simulink model "control_diagram_simple"  (R2018a)
settings: Solver=VariableStepAuto  StartTime=0.0  StopTime=10.0  RelTol=1e-3
libraries: fuzblock x2
settings Model: Creator=root  LastModifiedBy=User
settings DebuggingCC: LibraryContextMissingDiagnostic=warning
settings SFSimCC: SimUseLocalCustomCode=on
settings RTWCC: RTWUseLocalCustomCode=on

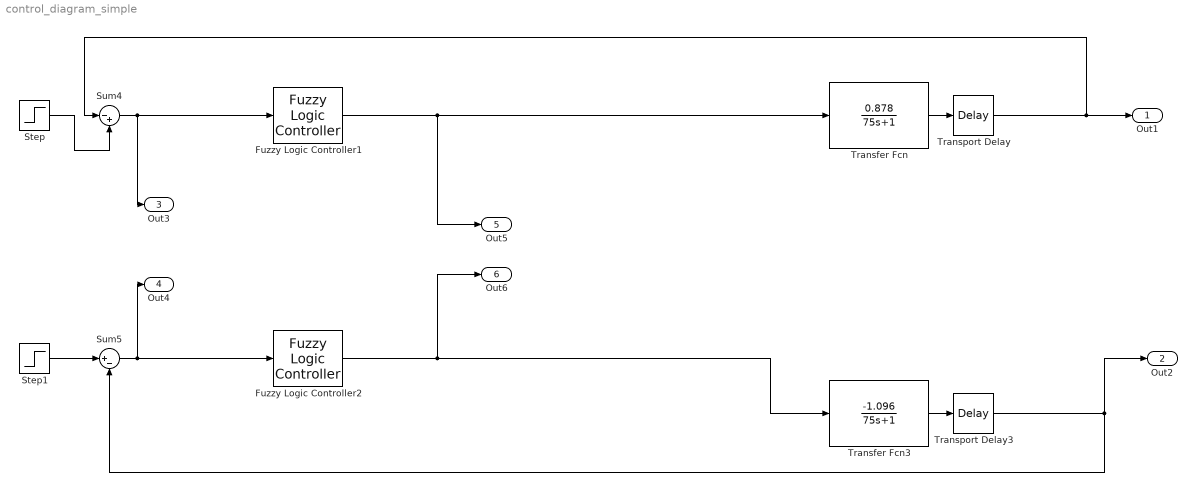
== system control_diagram_simple ==
  Fuzzy Logic Controller1 : fuzblock/Fuzzy Logic  Controller  FIS=flc1  OutputSampleNumber=101  DataType=double  FuzzifiedInputs=off  RuleFiringStrengths=off  RuleOutputs=off  AggregatedOutputs=off  SimulateUsing=Interpreted execution  OutOfRangeInputValueMessage=warning  NoRuleFiredMessage=warning  EmptyOutputFuzzySetMessage=warning
  Fuzzy Logic Controller2 : fuzblock/Fuzzy Logic  Controller  FIS=flc2  OutputSampleNumber=101  DataType=double  FuzzifiedInputs=off  RuleFiringStrengths=off  RuleOutputs=off  AggregatedOutputs=off  SimulateUsing=Interpreted execution  OutOfRangeInputValueMessage=warning  NoRuleFiredMessage=warning  EmptyOutputFuzzySetMessage=warning
  Step : Step  After=0.5  SampleTime=0
  Step1 : Step  After=0.5  SampleTime=0
  Sum4 : Sum  Inputs=|-+
  Sum5 : Sum  Inputs=|+-
  Transfer Fcn : TransferFcn  Numerator=[0.878]  Denominator=[75 1]
  Transfer Fcn3 : TransferFcn  Numerator=[-1.096]  Denominator=[75 1]
  Transport Delay : TransportDelay
  Transport Delay3 : TransportDelay
  Out1 : Outport  SignalName=y1
  Out2 : Outport  Port=2  SignalName=y2
  Out3 : Outport  Port=3  SignalName=Erro1
  Out4 : Outport  Port=4  SignalName=Erro2
  Out5 : Outport  Port=5  SignalName=Control1
  Out6 : Outport  Port=6  SignalName=Control2
  wires:
  Transfer Fcn/1 -> Transport Delay/1
  Transport Delay/1 -> Sum4/1, Out1/1
  Transfer Fcn3/1 -> Transport Delay3/1
  Fuzzy Logic Controller2/1 -> Out6/1, Transfer Fcn3/1
  Transport Delay3/1 -> Out2/1, Sum5/2
  Step/1 -> Sum4/2
  Sum4/1 -> Out3/1, Fuzzy Logic Controller1/1
  Step1/1 -> Sum5/1
  Sum5/1 -> Out4/1, Fuzzy Logic Controller2/1
  Fuzzy Logic Controller1/1 -> Out5/1, Transfer Fcn/1
